simulink model "balanceLQR"  (Simulink 8.1)
settings: Solver=ode3  SolverMode=SingleTasking  StartTime=0.0  StopTime=10.0  RelTol=1e-3
PreLoadFcn:
  | waijung.modelPreload; % Required for working with Waijung Blockset. Do not remove.
undefined symbols (not defined in the file or in its folder): ARM, DIR, disable_customio, enable_customio, in1, in2, inalpha, intheta, Link, LQFP100, MDK, out1, out2, output_customio, PD12, ST, STM32F407VG, STM32F4DISCOVERY
libraries: stm32f4_io_lib x2, waijung_customcode x1, stm32f4_device_config_lib x1
CloseFcn:
  | waijung.modelClose; % Required for working with Waijung Blockset. Do not remove.
settings Model: Creator=ThanhNhan  LastModifiedBy=ThanhNhan
settings DataIOCC: SignalLoggingSaveFormat=Dataset
settings OptimizationCC: ExpressionDepthLimit=128  OptimizeModelRefInitCode=on  LifeSpan=1
settings DebuggingCC: FcnCallInpInsideContextMsg=EnableAllAsError
settings HardwareCC: ProdEndianess=LittleEndian  ProdHWDeviceType=ARM Compatible->Cortex - M4  TargetEndianess=LittleEndian  TargetHWDeviceType=ARM Compatible->Cortex - M4
settings RTWCC: SystemTargetFile=stm32f4.tlc  GenerateMakefile=off  TemplateMakefile=ert_default_tmf  Description=STM32F4 Target  ProcessScript=stm32f4_make_rtw_hook
settings CodeAppCC: IgnoreCustomStorageClasses=off
settings STFCustomTargetCC: CodeReplacementLibrary=ANSI_C  ModelReferenceCompliant=off  CombineOutputUpdateFcns=on  ERTCustomFileBanners=on  SupportContinuousTime=off  SupportNonInlinedSFcns=off  MATLABClassNameForMDSCustomization=Simulink.SoftwareTarget.ERTCustomization  GRTInterface=off  SystemTargetFile=stm32f4.tlc
settings ERTTargetCC: CodeReplacementLibrary=ANSI_C  MultiwordLength=2048  ModelReferenceCompliant=off  ParMdlRefBuildCompliant=off  CompOptLevelCompliant=off  ConcurrentExecutionCompliant=off  ERTFirstTimeCompliant=off  ModelStepFunctionPrototypeControlCompliant=off  CPPClassGenCompliant=off  InlinedParameterPlacement=NonHierarchical  ERTSrcFileBannerTemplate=stm32f4_code_template.cgt  ERTHdrFileBannerTemplate=stm32f4_code_template.cgt  ERTDataSrcFileTemplate=stm32f4_code_template.cgt  ERTDataHdrFileTemplate=stm32f4_code_template.cgt  ERTCustomFileTemplate=stm32f4_file_process.tlc  ConvertIfToSwitch=off  SuppressUnreachableDefaultCases=off

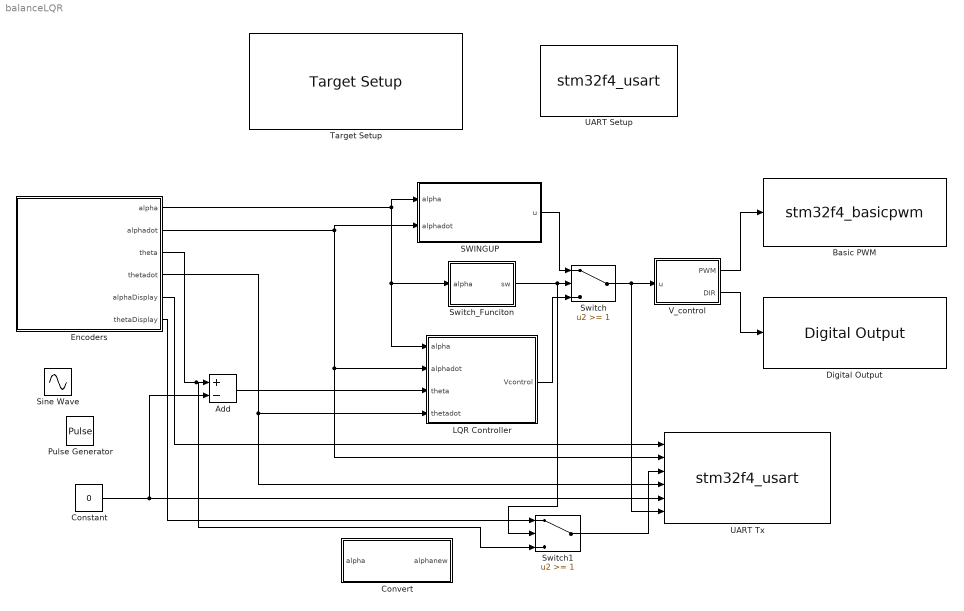
== system balanceLQR ==
  Add : Sum  Inputs=+-
  Basic PWM : S-Function  FunctionName=stm32f4_basicpwm  Parameters=timer,pwmperiod,ch1pin,ch2pin,ch3pin,ch4pin,sampletime,sampletimestr,blockid,apb,portstr,pinstr,pinmat,timarr,timprescale,chmat,polaritystr  EnableBusSupport=off  mask(stm32f4_basicpwm){timer=3, pwmperiod=0.00005, polarity=Active High, polaritystr=TIM_OCPolarity_High, ch1pin=A6, ch2pin=Not available - Do not use, ch3pin=Not available - Do not use, ch4pin=Not available - Do not use, sampletime=0.01, sampletimestr=0.01, blockid=BasicPWM, portpinstr=A6,,,, enablecustomportlabel=on, cinputportlabel=PWM_pulse, coutputportlabel=0, apb=1, portstr=["A"], pinstr=["GPIO_Pin_6"], pinmat=[1 6], timarr=4199, timprescale=0, chmat=[1]}
      mask prompts: pwmperiod "PWM Period (seconds)"; ch1pin "Channel 1"; ch2pin "Channel 2"; ch3pin "Channel 3"; ch4pin "Channel 4"; sampletime "Sample time (sec)"; sampletimestr "Compiled sample time (sec) in string"; portpinstr "Port pin string"; enablecustomportlabel "Enable custom port labels"; cinputportlabel "Custom input port labels (Ex. In1, In2, In3)"; coutputportlabel "Custom output port labels (Ex. Out1, Out2, Out3)"; portstr "Port string"; pinstr "Pin string"; pinmat "Pin matrix"; timarr "Timer ARR"; timprescale "Timer PRESCALE"; chmat "Channel order"
      mask help:
      | This block implements basic Edge-aligned Pulse Width Modulation (PWM) generation.
      | All timers are 16-bit. The PWM period is fixed (per timer).
      mask init:
      | stm32f4_basicpwm_callback('init');
      mask Help: web(fullfile(waijungdocroot,'stm32f4_basicpwm.htm'),'-browser')
      mask TypeOptions timer: 1 | 2 | 3 | 4 | 5 | 8 | 9 | 10 | 11 | 12 | 13 | 14
      mask Callback timer: stm32f4_basicpwm_callback('timer');
      mask Callback pwmperiod: stm32f4_basicpwm_callback('pwmperiod');
      mask TypeOptions polarity: Active High | Active Low
      mask Callback polarity: stm32f4_basicpwm_callback('polarity');
      mask TypeOptions ch1pin: Not available - Do not use | A6 | C6 | B4
      mask Callback ch1pin: stm32f4_basicpwm_callback('ch1pin');
      mask TypeOptions ch2pin: Not available - Do not use | A7 | C7 | B5
      mask Callback ch2pin: stm32f4_basicpwm_callback('ch2pin');
      mask TypeOptions ch3pin: Not available - Do not use | B0 | C8
      mask Callback ch3pin: stm32f4_basicpwm_callback('ch3pin');
      mask TypeOptions ch4pin: Not available - Do not use | B1 | C9
      mask Callback ch4pin: stm32f4_basicpwm_callback('ch4pin');
      mask Callback sampletime: stm32f4_basicpwm_callback('sampletime');
      mask Callback sampletimestr: stm32f4_basicpwm_callback('sampletimestr');
      mask Callback blockid: stm32f4_basicpwm_callback('blockid');
      mask Callback enablecustomportlabel: stm32f4_basicpwm_callback('enablecustomportlabel');
      mask Display: text(0.95, 0.5, 'Timer: 3\nPolarity: Active High\nPeriod (sec) 0.00005\nTs (sec): 0.01','ver','middle','hor','right');port_label('input', 1,'PWM_pulse (A6)')
  Constant : Constant  Value=0
  Convert : MATLAB Function  TreatAsAtomicUnit=on
  Digital Output : stm32f4_io_lib/Digital Output  use_bitband=on  port=D  speed=100  porttype=Push Pull  porttypestr=PP  use_pin0=off  use_pin1=off  use_pin2=off  use_pin3=off  use_pin4=off  use_pin5=off  use_pin6=off  use_pin7=off  use_pin8=off  use_pin9=off  use_pin10=off  use_pin11=off  use_pin12=on  use_pin13=off  use_pin14=off  use_pin15=off  pinstr=GPIO_Pin_12  usedpinarray="[0  0  0  0  0  0  0  0  0  0  0  0  1  0  0  0]"  bitbandingstr="#define DigitalOutput_D12 Peripheral_BB(GPIOD->ODR, 12)  /* Output pin */"  sampletime=-1  sampletimestr=0.01  blockid=DigitalOutput  enablecustomportlabel=on  cinputportlabel=DIR (PD12)  coutputportlabel=0
  Encoders : Subsystem
  LQR Controller : Subsystem
  Pulse Generator : DiscretePulseGenerator  PulseType=Time based  Amplitude=3  Period=20  PulseWidth=50
  SWINGUP : MATLAB Function  TreatAsAtomicUnit=on
  Sine Wave : Sin  Amplitude=1.3  Frequency=0.5  SampleTime=0.01
  Switch : Switch  Threshold=1
  Switch1 : Switch  Threshold=1
  Switch_Funciton : MATLAB Function  TreatAsAtomicUnit=on
  Target Setup : stm32f4_device_config_lib/Target Setup  Priority=100  compiler=MDK-ARM  mcu=STM32F407VG (LQFP100); STM32F4DISCOVERY  mcustr=STM32F407VG  clockconfig=STM32F4DISCOVERY Default (HSEOSC-8MHz/HCLK-168MHz)  system_stm32f4xx_c_path=E:\Learning\Matlab_Library_STM32F4\waijung13_10a\targets\stm32f4_target\stm32f4\utils\STM32F4xx_AN3988_V1.0.1\stm32f4_default\hseosc8mhz  showmemoryconfiguration=off  stacksize=0x2000  heapsize=0x2000  enableautocompiledownload=off  fullchiperase=off  programmerinterface=ST-Link  editctrlstr=off  compilercontrolstr=-c --cpu Cortex-M4.fp -g -O3 --apcs=interwork --split_sections $(INCLUDES)  assemblercontrolstr="--cpu Cortex-M4.fp -g --apcs=interwork  --xref $(INCLUDES)"  linkercontrolstr="--cpu Cortex-M4.fp --strict --scatter \"$(MODELNAME).sct\" --summary_stderr --info summarysizes --map --xref --callgraph --symbols --info sizes --info totals --info unused --info veneers  --list \".\\$(MODELNAME).map\" -o $(MODELNAME).axf"  runafterdownload=on  execprofile=None  profileruart=3  profilerbaud=500000  profilertxpin=D8  profilerinitstr=0.01,168000000,1680000,500000,0  manualsetsampletime=off  sampletime=0.01  blockid=TargetSetup  systickreloadvalue=1680000  hseval=8000000  lastprofileruart=3  hclk=168000000  flashorigin=0x8000000  flashlength=1M  ramorigin=0x20000000  ramlength=112k
  UART Setup : S-Function  Priority=1  FunctionName=stm32f4_usart  Parameters=configuration,uartmodule,transfer,baudrate,inputtype,outputtype,confstr,binheaderarray,binterminatorarray,asciiheader,asciiterminator,bindatalength,packetmode,varname,sampletime,sampletimestr,blockid  EnableBusSupport=off  mask(stm32f4_usart){configuration=Setup, uartmodule=1, baudrate=115200, databits=8, parity=No, stopbit=1, remaptxpin=B6, remaprxpin=B7, flowcontrol=None, remapctspin=Not used, remaprtspin=Not used, advanceoptions=off, rxbuffersize=512, txbuffersize=512, transfer=Blocking, packetmode=Ascii, binheader='7E 7E', binterminator='03 03', porttype_double=1, porttype_single=0, porttype_int8=1, porttype_uint8=0, porttype_int16=0, porttype_uint16=0, porttype_int32=0, porttype_uint32=0, asciiformat='%d,%f', rx_asciiterminator=CRLF (0x0D 0x0A - "\r\n"), tx_asciiterminator=CR (0x0D - "\r"), storagename=<empty>, varname=, inputtype=[0], outputtype=[0], binheaderarray=[0], binterminatorarray=[0], bindatalength=0, asciiheader='', asciiterminator=[0], sampletime=inf, sampletimestr=0.01, blockid=UARTSetup, confstr=[ "dummy", "1", "B", "6", "1", "B", "7", "0", "*", "*", "0", "*", "*", "2", "4", "7", "2", "4", "2", "512", "512", "2", "1", "115200", "8", "No", "1", "None", "USART1"], lastmodule=1}
      mask prompts: uartmodule "UART Module"; baudrate "Baud rate (bps)"; databits "Data bits"; stopbit "Stop bit"; remaptxpin "Tx Pin"; remaprxpin "Rx Pin"; flowcontrol "Hardware flow control"; remapctspin "HW Flow control, CTS Pin"; remaprtspin "HW Flow control, RTS Pin"; advanceoptions "Advance options"; rxbuffersize "Rx buffer size (bytes)"; txbuffersize "Tx buffer size (bytes)"; packetmode "Packet mode"; binheader "Binary header (example: '7E 7E')"; binterminator "Binary terminator (example: '03 03')"; porttype_double "Number of data port, type DOUBLE"; porttype_single "Number of data port, type SINGLE"; porttype_int8 "Number of data port, type INT8"; porttype_uint8 "Number of data port, type UINT8"; porttype_int16 "Number of data port, type INT16"; porttype_uint16 "Number of data port, type UINT16"; porttype_int32 "Number of data port, type INT32"; porttype_uint32 "Number of data port, type UINT32"; asciiformat "Ascii format"; rx_asciiterminator "End of packet"; tx_asciiterminator "End of packet"; storagename "Buffer"; varname "Var name"; inputtype "Input data type"; outputtype "Output data type"; binheaderarray "Binary header"; binterminatorarray "Binary terminator"; bindatalength "Binary data length"; asciiheader "Ascii header (printf format)"; asciiterminator "Ascii terminator"; sampletime "Sample time (sec)"; sampletimestr "Compiled sample time (sec) in string"; confstr "Configuration string"; lastmodule "Last module selected"
      mask help:
      | Default STM32F4DISCOVERY + aMG F4 Connect 2 + aMG USB Converter N2 settings use
      |
      | USART3, Tx D8, Rx D9 and USB Serial Converter A.
      mask init:
      | stm32f4_usart_callback('init');
      mask Help: web(fullfile(waijungdocroot,'stm32f4_usart_setup.htm'), '-browser')
      mask TypeOptions configuration: Setup | Tx | Rx
      mask Callback configuration: stm32f4_usart_callback('configuration');
      mask TypeOptions uartmodule: 1 | 2 | 3 | 4 | 5 | 6
      mask Callback uartmodule: stm32f4_usart_callback('uartmodule');
      mask Callback baudrate: stm32f4_usart_callback('baudrate');
      mask TypeOptions databits: 8
      mask TypeOptions parity: No | Odd | Even
      mask TypeOptions stopbit: 0.5 | 1 | 1.5 | 2
      mask TypeOptions remaptxpin: Not used | A9 | B6
      mask TypeOptions remaprxpin: Not used | A10 | B7
      mask TypeOptions flowcontrol: None | RTS | CTS | RTS/CTS
      mask Callback flowcontrol: stm32f4_usart_callback('flowcontrol');
      mask TypeOptions remapctspin: Not used | A11
      mask TypeOptions remaprtspin: Not used | A12
      mask Callback advanceoptions: stm32f4_usart_callback('advanceoptions');
      mask TypeOptions rxbuffersize: 16 | 32 | 64 | 128 | 256 | 512 | 1024 | 2048
      mask TypeOptions txbuffersize: 16 | 32 | 64 | 128 | 256 | 512 | 1024 | 2048
      mask TypeOptions transfer: Blocking | Non-Blocking
      mask Callback transfer: stm32f4_usart_callback('transfer');
      mask TypeOptions packetmode: Ascii | Binary | String Buffer
      mask Callback packetmode: stm32f4_usart_callback('packetmode');
      mask Callback binheader: stm32f4_usart_callback('binheader');
      mask Callback binterminator: stm32f4_usart_callback('binterminator');
      mask Callback porttype_double: stm32f4_usart_callback('porttype');
      mask Callback porttype_single: stm32f4_usart_callback('porttype');
      mask Callback porttype_int8: stm32f4_usart_callback('porttype');
      mask Callback porttype_uint8: stm32f4_usart_callback('porttype');
      mask Callback porttype_int16: stm32f4_usart_callback('porttype');
      mask Callback porttype_uint16: stm32f4_usart_callback('porttype');
      mask Callback porttype_int32: stm32f4_usart_callback('porttype');
      mask Callback porttype_uint32: stm32f4_usart_callback('porttype');
      mask Callback asciiformat: stm32f4_usart_callback('asciiformat');
      mask TypeOptions rx_asciiterminator: CR (0x0D - "\r") | LF (0x0A - "\n") | CRLF (0x0D 0x0A - "\r\n")
      mask Callback rx_asciiterminator: stm32f4_usart_callback('rx_asciiterminator');
      mask TypeOptions tx_asciiterminator: CR (0x0D - "\r") | LF (0x0A - "\n") | CRLF (0x0D 0x0A - "\r\n") | None
      mask Callback tx_asciiterminator: stm32f4_usart_callback('tx_asciiterminator');
      mask TypeOptions storagename: <empty>
      mask Callback storagename: stm32f4_usart_callback('storagename');
      mask Callback varname: stm32f4_usart_callback('varname');
      mask Callback sampletime: stm32f4_usart_callback('sampletime');
      mask Callback sampletimestr: stm32f4_usart_callback('sampletimestr');
      mask Callback blockid: stm32f4_usart_callback('blockid');
      mask Display: text(0.5, 0.5, 'Module: USART1_Setup\nBaud (Bps): 115200\nDMA Buffer: 512/512\nTx/Rx Pin: B6/B7','ver','middle','hor','center');
  UART Tx : S-Function  Priority=1  FunctionName=stm32f4_usart  Parameters=configuration,uartmodule,transfer,baudrate,inputtype,outputtype,confstr,binheaderarray,binterminatorarray,asciiheader,asciiterminator,bindatalength,packetmode,varname,sampletime,sampletimestr,blockid  EnableBusSupport=off  mask(stm32f4_usart){configuration=Tx, uartmodule=1, baudrate=115200, databits=8, parity=No, stopbit=1, remaptxpin=Not used, remaprxpin=Not used, flowcontrol=None, remapctspin=Not used, remaprtspin=Not used, advanceoptions=off, rxbuffersize=512, txbuffersize=512, transfer=Blocking, packetmode=Binary, binheader='7E 7E', binterminator='03 03', porttype_double=6, porttype_single=0, porttype_int8=0, porttype_uint8=0, porttype_int16=0, porttype_uint16=0, porttype_int32=0, porttype_uint32=0, asciiformat='value=%d,%f', rx_asciiterminator=CRLF (0x0D 0x0A - "\r\n"), tx_asciiterminator=CRLF (0x0D 0x0A - "\r\n"), storagename=<empty>, varname=, inputtype=[6  0 0 0 0 0 0], outputtype=[0], binheaderarray=[2 126  126], binterminatorarray=[2 3  3], bindatalength=48, asciiheader='value=%d,%f\r\n', asciiterminator=[2 13 10], sampletime=-1, sampletimestr=0.01, blockid=UARTTx, confstr=[ "dummy", "0", "*", "*", "0", "*", "*", "0", "*", "*", "0", "*", "*", "2", "4", "7", "2", "4", "2", "512", "512", "2", "1", "115200", "8", "No", "1", "None", "USART1"], lastmodule=1}
      mask prompts: uartmodule "UART Module"; baudrate "Baud rate (bps)"; databits "Data bits"; stopbit "Stop bit"; remaptxpin "Tx Pin"; remaprxpin "Rx Pin"; flowcontrol "Hardware flow control"; remapctspin "HW Flow control, CTS Pin"; remaprtspin "HW Flow control, RTS Pin"; advanceoptions "Advance options"; rxbuffersize "Rx buffer size (bytes)"; txbuffersize "Tx buffer size (bytes)"; packetmode "Packet mode"; binheader "Binary header (example: '7E 7E')"; binterminator "Binary terminator (example: '03 03')"; porttype_double "Number of data port, type DOUBLE"; porttype_single "Number of data port, type SINGLE"; porttype_int8 "Number of data port, type INT8"; porttype_uint8 "Number of data port, type UINT8"; porttype_int16 "Number of data port, type INT16"; porttype_uint16 "Number of data port, type UINT16"; porttype_int32 "Number of data port, type INT32"; porttype_uint32 "Number of data port, type UINT32"; asciiformat "Ascii format"; rx_asciiterminator "End of packet"; tx_asciiterminator "End of packet"; storagename "Buffer"; varname "Var name"; inputtype "Input data type"; outputtype "Output data type"; binheaderarray "Binary header"; binterminatorarray "Binary terminator"; bindatalength "Binary data length"; asciiheader "Ascii header (printf format)"; asciiterminator "Ascii terminator"; sampletime "Sample time (sec)"; sampletimestr "Compiled sample time (sec) in string"; confstr "Configuration string"; lastmodule "Last module selected"
      mask help:
      | Data type for Ascii format
      | %u, %i, %d, %o, %x: uint32
      | %e, %g, %f: single
      | %c: int8
      mask init:
      | stm32f4_usart_callback('init');
      mask Help: web(fullfile(waijungdocroot,'stm32f4_usart_tx.htm'), '-browser')
      mask TypeOptions configuration: Setup | Tx | Rx
      mask Callback configuration: stm32f4_usart_callback('configuration');
      mask TypeOptions uartmodule: 1 | 2 | 3 | 4 | 5 | 6
      mask Callback uartmodule: stm32f4_usart_callback('uartmodule');
      mask Callback baudrate: stm32f4_usart_callback('baudrate');
      mask TypeOptions databits: 8
      mask TypeOptions parity: No | Odd | Even
      mask TypeOptions stopbit: 0.5 | 1 | 1.5 | 2
      mask TypeOptions remaptxpin: Not used | A9 | B6
      mask TypeOptions remaprxpin: Not used | A10 | B7
      mask TypeOptions flowcontrol: None | RTS | CTS | RTS/CTS
      mask Callback flowcontrol: stm32f4_usart_callback('flowcontrol');
      mask TypeOptions remapctspin: Not used | A11
      mask TypeOptions remaprtspin: Not used | A12
      mask Callback advanceoptions: stm32f4_usart_callback('advanceoptions');
      mask TypeOptions rxbuffersize: 16 | 32 | 64 | 128 | 256 | 512 | 1024 | 2048
      mask TypeOptions txbuffersize: 16 | 32 | 64 | 128 | 256 | 512 | 1024 | 2048
      mask TypeOptions transfer: Blocking | Non-Blocking
      mask Callback transfer: stm32f4_usart_callback('transfer');
      mask TypeOptions packetmode: Ascii | Binary | String Buffer
      mask Callback packetmode: stm32f4_usart_callback('packetmode');
      mask Callback binheader: stm32f4_usart_callback('binheader');
      mask Callback binterminator: stm32f4_usart_callback('binterminator');
      mask Callback porttype_double: stm32f4_usart_callback('porttype');
      mask Callback porttype_single: stm32f4_usart_callback('porttype');
      mask Callback porttype_int8: stm32f4_usart_callback('porttype');
      mask Callback porttype_uint8: stm32f4_usart_callback('porttype');
      mask Callback porttype_int16: stm32f4_usart_callback('porttype');
      mask Callback porttype_uint16: stm32f4_usart_callback('porttype');
      mask Callback porttype_int32: stm32f4_usart_callback('porttype');
      mask Callback porttype_uint32: stm32f4_usart_callback('porttype');
      mask Callback asciiformat: stm32f4_usart_callback('asciiformat');
      mask TypeOptions rx_asciiterminator: CR (0x0D - "\r") | LF (0x0A - "\n") | CRLF (0x0D 0x0A - "\r\n")
      mask Callback rx_asciiterminator: stm32f4_usart_callback('rx_asciiterminator');
      mask TypeOptions tx_asciiterminator: CR (0x0D - "\r") | LF (0x0A - "\n") | CRLF (0x0D 0x0A - "\r\n") | None
      mask Callback tx_asciiterminator: stm32f4_usart_callback('tx_asciiterminator');
      mask TypeOptions storagename: <empty>
      mask Callback storagename: stm32f4_usart_callback('storagename');
      mask Callback varname: stm32f4_usart_callback('varname');
      mask Callback sampletime: stm32f4_usart_callback('sampletime');
      mask Callback sampletimestr: stm32f4_usart_callback('sampletimestr');
      mask Callback blockid: stm32f4_usart_callback('blockid');
      mask Display: text(0.95, 0.5, 'Module: USART1_Tx\nPacket: Binary\nTransfer: Blocking\nTs (sec): 0.01','ver','middle','hor','right'); port_label('input', 1,'double'); port_label('input', 2,'double'); port_label('input', 3,'double'); port_label('input', 4,'double'); port_label('input', 5,'double'); port_label('input', 6,'double');
  V_control : MATLAB Function  TreatAsAtomicUnit=on
  wires:
  Encoders/1(alpha) -> SWINGUP/1(alpha), LQR Controller/1(alpha), Switch_Funciton/1(alpha)
  V_control/1(PWM) -> Basic PWM/1
  V_control/2(DIR) -> Digital Output/1
  Switch/1 -> UART Tx/6, V_control/1(u)
  SWINGUP/1(u) -> Switch/1
  Switch_Funciton/1(sw) -> Switch1/2, Switch/2
  Encoders/4(thetadot) -> UART Tx/4, LQR Controller/4(thetadot)
  Add/1 -> LQR Controller/3(theta)
  Encoders/2(alphadot) -> UART Tx/2, LQR Controller/2(alphadot), SWINGUP/2(alphadot)
  Encoders/3(theta) -> Switch1/3, Add/1
  LQR Controller/1(Vcontrol) -> Switch/3
  Constant/1 -> Add/2, UART Tx/5
  Encoders/5(alphaDisplay) -> UART Tx/1
  Encoders/6(thetaDisplay) -> Switch1/1
  Switch1/1 -> UART Tx/3

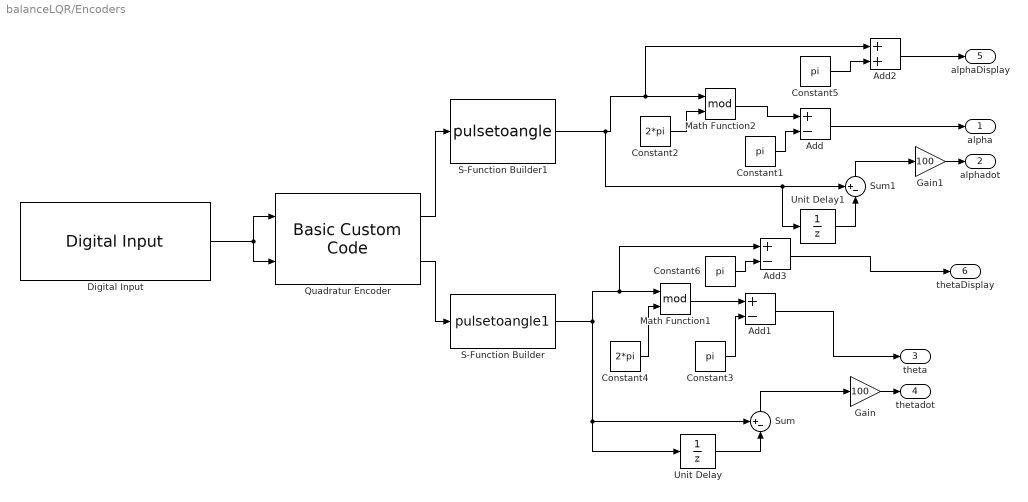
== system balanceLQR/Encoders ==
  Add : Sum  Inputs=+-
  Add1 : Sum  Inputs=+-
  Add2 : Sum
  Add3 : Sum  Inputs=+-
  Constant{1,3,5..6} (4 alike) : Constant  Value=pi
  Constant2 : Constant  Value=2*pi
  Constant4 : Constant  Value=2*pi
  Digital Input : stm32f4_io_lib/Digital Input  port=A  speed=100  porttype=None  porttypestr=NOPULL  use_pin0=on  use_pin1=off  use_pin2=off  use_pin3=off  use_pin4=off  use_pin5=off  use_pin6=off  use_pin7=off  use_pin8=off  use_pin9=off  use_pin10=off  use_pin11=off  use_pin12=off  use_pin13=off  use_pin14=off  use_pin15=off  pinstr=GPIO_Pin_0  usedpinarray="[1  0  0  0  0  0  0  0  0  0  0  0  0  0  0  0]"  bitbandingstr="#define EncodersDigitalInput_A0 Peripheral_BB(GPIOA->IDR, 0)  /* Output pin */"  sampletime=0.01  sampletimestr=0.01  blockid=EncodersDigitalInput  enablecustomportlabel=off  cinputportlabel=In1, In2  coutputportlabel=Out1, Out2
  Gain : Gain  Gain=100
  Gain1 : Gain  Gain=100
  Math Function1 : Math  Operator=mod  SaturateOnIntegerOverflow=on
  Math Function2 : Math  Operator=mod  SaturateOnIntegerOverflow=on
  Quadratur Encoder : waijung_customcode/Basic Custom Code  inputporttype=boolean,boolean  cinputportlabel=inalpha,intheta  cinputportlabelstr="[\"inalpha\",\"intheta\"]"  inputportcount=2  inputporttypeid="[8  8]"  outputporttype=int32,int32  coutputportlabel=alpha, theta  coutputportlabelstr="[\"alpha\",\" theta\"]"  outputportcount=2  outputporttypeid="[6  6]"  incpath={fullfile(pwd,'customcode')}  srcpath={fullfile(pwd,'customcode')}  incfiles={'stm32f4_io_customcode.h'}  srcfiles={'stm32f4_io_customcode.c'}  enablefuncallstr=enable_customio();  outputfuncallstr=output_customio(in1,in2,out1,out2);  disablefuncallstr=disable_customio();  sampletime=-1  sampletimestr=0.01  blockid=EncodersQuadraturEncoder  enablecustomportlabel=on  incfilestrarray="[\"stm32f4_io_customcode.h\"]"
  S-Function Builder : S-Function  InitFcn=try, set_param(gcb,'FunctionName','pulsetoangle1'), end  FunctionName=pulsetoangle1  SFunctionModules=pulsetoangle1_wrapper  WizardData=DataTag0  EnableBusSupport=off  mask(S-Function Builder){}
      mask help: Simulink:masks:SFunctionBuilder_MD
      mask init:
      | val = [[.9  0.75 0.75 1 1 .9 .9 1]',[1 1 0.75 0.75 .9 .9 1 .9]'];try , sys = get_param(gcb,'SfunBuilderFcnName');if isempty(sys), sys = get_param(gcb,'FunctionName'); end,catch, sys = get_param(gcb,'FunctionName'); end
      settings: CopyFcn=set_param(gcbh,'LinkStatus','none')  PreSaveFcn=try, set_param(gcb,'FunctionName','pulsetoangle1'), end  OpenFcn=sfunctionwizard(gcbh)
      mask Display: plot(val(:,1),val(:,2)),disp(sys), port_label('input',1,'u0'), port_label('output',1,'y0')
  S-Function Builder1 : S-Function  InitFcn=try, set_param(gcb,'FunctionName','pulsetoangle'), end  FunctionName=pulsetoangle  SFunctionModules=pulsetoangle_wrapper  WizardData=DataTag1  EnableBusSupport=off  mask(S-Function Builder){}
      mask help: Simulink:masks:SFunctionBuilder_MD
      mask init: same as balanceLQR/Encoders/S-Function Builder
      settings: CopyFcn=set_param(gcbh,'LinkStatus','none')  PreSaveFcn=try, set_param(gcb,'FunctionName','pulsetoangle'), end  OpenFcn=sfunctionwizard(gcbh)
      mask Display: plot(val(:,1),val(:,2)),disp(sys), port_label('input',1,'u0'), port_label('output',1,'y0')
  Sum : Sum  Inputs=+-|
  Sum1 : Sum  Inputs=+-|
  Unit Delay : UnitDelay  SampleTime=-1
  Unit Delay1 : UnitDelay  SampleTime=-1
  alpha : Outport
  alphadot : Outport  Port=2
  theta : Outport  Port=3
  thetadot : Outport  Port=4
  alphaDisplay : Outport  Port=5
  thetaDisplay : Outport  Port=6
  wires:
  S-Function Builder/1 -> Unit Delay/1, Sum/1, Add3/1, Math Function1/1
  Quadratur Encoder/2 -> S-Function Builder/1
  Sum/1 -> Gain/1
  Gain/1 -> thetadot/1
  Unit Delay/1 -> Sum/2
  Quadratur Encoder/1 -> S-Function Builder1/1
  Sum1/1 -> Gain1/1
  Gain1/1 -> alphadot/1
  Unit Delay1/1 -> Sum1/2
  Digital Input/1 -> Quadratur Encoder/1, Quadratur Encoder/2
  Constant1/1 -> Add/2
  Constant3/1 -> Add1/2
  Constant4/1 -> Math Function1/2
  Constant2/1 -> Math Function2/2
  S-Function Builder1/1 -> Sum1/1, Unit Delay1/1, Add2/1, Math Function2/1
  Math Function2/1 -> Add/1
  Add1/1 -> theta/1
  Add/1 -> alpha/1
  Add2/1 -> alphaDisplay/1
  Constant5/1 -> Add2/2
  Math Function1/1 -> Add1/1
  Constant6/1 -> Add3/2
  Add3/1 -> thetaDisplay/1

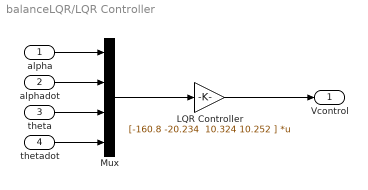
== system balanceLQR/LQR Controller ==
  alpha : Inport
  alphadot : Inport  Port=2
  theta : Inport  Port=3
  thetadot : Inport  Port=4
  LQR Controller : Gain  Gain="[-160.8 -20.234  10.324 10.252 ]"  Multiplication=Matrix(K*u)
  Mux : Mux
  Vcontrol : Outport
  wires:
  Mux/1 -> LQR Controller/1
  LQR Controller/1 -> Vcontrol/1
  alpha/1 -> Mux/1
  alphadot/1 -> Mux/2
  theta/1 -> Mux/3
  thetadot/1 -> Mux/4

== matlab function V_control ==
  data: u input double; PWM output double; DIR output double
function [PWM, DIR] = fcn(u)
%#codegen
if u<0
    DIR=0;
    PWM=-u*100/24;
else
%     DIR=1;
%     PWM=u*100/24;
DIR=1;
PWM=u*100/24;

end

== matlab function SWINGUP ==
  data: u output double; alpha input double; alphadot input double
%#************************
%energy based control
%#***********************88

function u = SWING_UP(alpha,alphadot)
%if (alpha>0.6)||(alpha<-0.6)
voltage=5;
if (alphadot*cos(alpha))<0
    u=-voltage;
% % % % % % elseif (alphadot*cos(alpha))>0
% % % % % %     u=voltage;
% if(q1>pi)&&(q1<2*pi)
%     q1=q1-2*pi;
% if(abs(q2)<pi/2)
% if((alpha>=pi)&&(alpha<3*pi/2)&&(alphadot<=0))
%     u=20;
% elseif ((alpha<pi)&&(alpha>pi/2)&&(alphadot>0))
%     u=-20;
% % if((alpha>=-pi)&&(alpha<-pi/2)&&(alphadot<=0))
% %     u=10;
% % elseif ((alpha<pi)&&(alpha>pi/2)&&(alphadot>0))
% %     u=-10;
% elseif ((abs(q1)< pi/18))
%     u = -(q2*(-10)+ q1*(53.5434) + q2dot*(-4.9882) + q1dot*(7.4922));
% else
%     u = 0;
% end
% elseif(q2>pi)
%     u=-3;
else
    u=voltage;
end
%else u=0;
end



% if u >=24
%     u = 24;
% end
% if u <= -24
%     u = -24;
% end -10.0000   53.5434   -4.9882    7.4922

== matlab function Switch_Funciton ==
  data: alpha input double; sw output double
function sw = Switch(alpha)
if (alpha<0.314)&&(alpha>-0.314)
    sw = 0;
else
    sw = 1;
end

== matlab function Convert ==
  data: alpha input double; alphanew output double
function alphanew = convert(alpha)
if (alpha>=pi)
    alphanew=alpha-pi;
else
    alphanew=alpha+pi;
end
